simulink model "main"  (R2022a)
settings: Solver=FixedStepDiscrete  StartTime=0.0  StopTime=Inf  FixedStep=(50e-6)-(sim_en*4.995e-5)  RelTol=1e-3  EnableMultiTasking=on
model workspace (MAT data in the model file):
  Param : Simulink.Parameter (value not decoded)
  ac_ok : Simulink.Signal (value not decoded)
  ac_ok_120 : Simulink.Signal (value not decoded)
  bulk_voltage : Simulink.Signal (value not decoded)
  burstduty_integ_max : Simulink.Signal (value not decoded)
  burstduty_integ_min : Simulink.Signal (value not decoded)
  burstduty_ki : Simulink.Signal (value not decoded)
  burstduty_kp : Simulink.Signal (value not decoded)
  calib_ok : Simulink.Signal (value not decoded)
  can_addr1 : Simulink.Signal (value not decoded)
  can_addr2 : Simulink.Signal (value not decoded)
  can_addr3 : Simulink.Signal (value not decoded)
  can_addr4 : Simulink.Signal (value not decoded)
  can_data_rx : Simulink.Signal (value not decoded)
  can_data_tx : Simulink.Signal (value not decoded)
  can_timeout_120 : Simulink.Signal (value not decoded)
  chksum_scircv : Simulink.Signal (value not decoded)
  clllc_en_120 : Simulink.Signal (value not decoded)
  clllc_fault_120 : Simulink.Signal (value not decoded)
  clllc_ok_120 : Simulink.Signal (value not decoded)
  cmpss1h : Simulink.Signal (value not decoded)
  cmpss1l : Simulink.Signal (value not decoded)
  cmpss2h : Simulink.Signal (value not decoded)
  cmpss2l : Simulink.Signal (value not decoded)
  cmpss3h : Simulink.Signal (value not decoded)
  cmpss3l : Simulink.Signal (value not decoded)
  cmpss4h : Simulink.Signal (value not decoded)
  cmpss4l : Simulink.Signal (value not decoded)
  cmpss5h : Simulink.Signal (value not decoded)
  cmpss5l : Simulink.Signal (value not decoded)
  cmpss6h : Simulink.Signal (value not decoded)
  cmpss6l : Simulink.Signal (value not decoded)
  cmpss7h : Simulink.Signal (value not decoded)
  cmpss7l : Simulink.Signal (value not decoded)
  cmpss8h : Simulink.Signal (value not decoded)
  cmpss8l : Simulink.Signal (value not decoded)
  cnt_idle : Simulink.Signal (value not decoded)
  cnt_orps : Simulink.Signal (value not decoded)
  cnt_scircv : Simulink.Signal (value not decoded)
  cnt_scixmt : Simulink.Signal (value not decoded)
  cnt_scixmt_func : Simulink.Signal (value not decoded)
  cnt_temp_mux : Simulink.Signal (value not decoded)
  cnt_vdroop : Simulink.Signal (value not decoded)
  config_ok : Simulink.Signal (value not decoded)
  control_en : Simulink.Signal (value not decoded)
  cp_ready_120 : Simulink.Signal (value not decoded)
  d2d_en : Simulink.Signal (value not decoded)
  dchg_off : Simulink.Signal (value not decoded)
  debug_dacb : Simulink.Signal (value not decoded)
  debug_dacc : Simulink.Signal (value not decoded)
  debug_msg1 : Simulink.Signal (value not decoded)
  debug_msg2 : Simulink.Signal (value not decoded)
  debug_msg3 : Simulink.Signal (value not decoded)
  debug_msg4 : Simulink.Signal (value not decoded)
  debug_msg5 : Simulink.Signal (value not decoded)
  debug_msg6 : Simulink.Signal (value not decoded)
  dir_v2g : Simulink.Signal (value not decoded)
  eoss_llc1 : Simulink.Signal (value not decoded)
  eoss_llc2 : Simulink.Signal (value not decoded)
  eoss_orps : Simulink.Signal (value not decoded)
  fault_ocp : Simulink.Signal (value not decoded)
  fault_otp : Simulink.Signal (value not decoded)
  fault_ovp : Simulink.Signal (value not decoded)
  fut_en : Simulink.Signal (value not decoded)
  fwd_en_120 : Simulink.Signal (value not decoded)
  gain_llc1_sec_idc : Simulink.Signal (value not decoded)
  gain_llc1_temp_sr : Simulink.Signal (value not decoded)
  gain_llc2_sec_idc : Simulink.Signal (value not decoded)
  gain_vbat : Simulink.Signal (value not decoded)
  gain_vbulk : Simulink.Signal (value not decoded)
  gain_vout : Simulink.Signal (value not decoded)
  input_current_phasea : Simulink.Signal (value not decoded)
  input_current_phaseb : Simulink.Signal (value not decoded)
  input_current_phasec : Simulink.Signal (value not decoded)
  input_freq : Simulink.Signal (value not decoded)
  input_power : Simulink.Signal (value not decoded)
  input_voltage_phasea : Simulink.Signal (value not decoded)
  input_voltage_phaseb : Simulink.Signal (value not decoded)
  input_voltage_phasec : Simulink.Signal (value not decoded)
  ishare_arbiter : Simulink.Signal (value not decoded)
  ishare_thresh : Simulink.Signal (value not decoded)
  led_g : Simulink.Signal (value not decoded)
  led_r : Simulink.Signal (value not decoded)
  led_y : Simulink.Signal (value not decoded)
  llc1_burst_integ : Simulink.Signal (value not decoded)
  llc1_burstduty_buffer : Simulink.Signal (value not decoded)
  llc1_pfm_error : Simulink.Signal (value not decoded)
  llc1_pfm_integ : Simulink.Signal (value not decoded)
  llc1_pfm_prop : Simulink.Signal (value not decoded)
  llc1_pri_idc : Simulink.Signal (value not decoded)
  llc1_ps_buffer : Simulink.Signal (value not decoded)
  llc1_pspwm_error : Simulink.Signal (value not decoded)
  llc1_pspwm_integ : Simulink.Signal (value not decoded)
  llc1_pspwm_prop : Simulink.Signal (value not decoded)
  llc1_sec_idc : Simulink.Signal (value not decoded)
  llc1_temp_sr : Simulink.Signal (value not decoded)
  llc1_ts_tbctr_buffer : Simulink.Signal (value not decoded)
  llc2_burst_integ : Simulink.Signal (value not decoded)
  llc2_burstduty_buffer : Simulink.Signal (value not decoded)
  llc2_en : Simulink.Signal (value not decoded)
  llc2_en_buffer : Simulink.Signal (value not decoded)
  llc2_pfm_error : Simulink.Signal (value not decoded)
  llc2_pfm_integ : Simulink.Signal (value not decoded)
  llc2_pfm_prop : Simulink.Signal (value not decoded)
  llc2_pri_idc : Simulink.Signal (value not decoded)
  llc2_ps_buffer : Simulink.Signal (value not decoded)
  llc2_pspwm_error : Simulink.Signal (value not decoded)
  llc2_pspwm_integ : Simulink.Signal (value not decoded)
  llc2_pspwm_prop : Simulink.Signal (value not decoded)
  llc2_sec_idc : Simulink.Signal (value not decoded)
  llc2_temp_sr : Simulink.Signal (value not decoded)
  llc2_ts_tbctr_buffer : Simulink.Signal (value not decoded)
  loop_adcint : Simulink.Signal (value not decoded)
  loop_control : Simulink.Signal (value not decoded)
  loop_idle : Simulink.Signal (value not decoded)
  mid_bulk_voltage : Simulink.Signal (value not decoded)
  mode_120 : Simulink.Signal (value not decoded)
  mode_cc_cv : Simulink.Signal (value not decoded)
  myParam : mpt.Parameter (value not decoded)
  obc_ok_120 : Simulink.Signal (value not decoded)
  offset_llc1_sec_idc : Simulink.Signal (value not decoded)
  offset_llc1_temp_sr : Simulink.Signal (value not decoded)
  offset_llc2_sec_idc : Simulink.Signal (value not decoded)
  offset_vbat : Simulink.Signal (value not decoded)
  offset_vbulk : Simulink.Signal (value not decoded)
  offset_vout : Simulink.Signal (value not decoded)
  openloop_en : Simulink.Signal (value not decoded)
  openloop_fault_en : Simulink.Signal (value not decoded)
  ot_fault_120 : Simulink.Signal (value not decoded)
  pfc_en : Simulink.Signal (value not decoded)
  pfc_en_120 : Simulink.Signal (value not decoded)
  pfc_fw_revision : Simulink.Signal (value not decoded)
  pfc_fw_revision_bootloader : Simulink.Signal (value not decoded)
  pfc_fw_revision_debug : Simulink.Signal (value not decoded)
  pfc_ok : Simulink.Signal (value not decoded)
  pfc_ok_120 : Simulink.Signal (value not decoded)
  pfm_a0 : Simulink.Signal (value not decoded)
  pfm_a1 : Simulink.Signal (value not decoded)
  pfm_integ_max : Simulink.Signal (value not decoded)
  pfm_integ_min : Simulink.Signal (value not decoded)
  pfm_ki : Simulink.Signal (value not decoded)
  pfm_kp : Simulink.Signal (value not decoded)
  pri_fut_en : Simulink.Signal (value not decoded)
  pri_fut_en_buffer : Simulink.Signal (value not decoded)
  pri_halfbridge_en : Simulink.Signal (value not decoded)
  pri_halfbridge_en_buffer : Simulink.Signal (value not decoded)
  pspwm_integ_max : Simulink.Signal (value not decoded)
  pspwm_integ_min : Simulink.Signal (value not decoded)
  pspwm_ki : Simulink.Signal (value not decoded)
  pspwm_kp : Simulink.Signal (value not decoded)
  ref_idclink_max : Simulink.Signal (value not decoded)
  ref_iout : Simulink.Signal (value not decoded)
  ref_iout_calib : Simulink.Signal (value not decoded)
  ref_iout_llc1 : Simulink.Signal (value not decoded)
  ref_iout_llc1_calib : Simulink.Signal (value not decoded)
  ref_iout_llc2 : Simulink.Signal (value not decoded)
  ref_iout_llc2_calib : Simulink.Signal (value not decoded)
  ref_pout : Simulink.Signal (value not decoded)
  ref_ss_llc1 : Simulink.Signal (value not decoded)
  ref_ss_llc2 : Simulink.Signal (value not decoded)
  ref_ss_orps : Simulink.Signal (value not decoded)
  ref_vbat : Simulink.Signal (value not decoded)
  ref_vbat_calib : Simulink.Signal (value not decoded)
  ref_vbulk : Simulink.Signal (value not decoded)
  ref_vbulk_calib : Simulink.Signal (value not decoded)
  ref_vbulk_llc1_calib : Simulink.Signal (value not decoded)
  ref_vbulk_llc2_calib : Simulink.Signal (value not decoded)
  ref_vout : Simulink.Signal (value not decoded)
  ref_vout_calib : Simulink.Signal (value not decoded)
  relay_en : Simulink.Signal (value not decoded)
  reset_flag : Simulink.Signal (value not decoded)
  rev_en_120 : Simulink.Signal (value not decoded)
  runtime_control : Simulink.Signal (value not decoded)
  runtime_idle : Simulink.Signal (value not decoded)
  scircv_buffer : Simulink.Signal (value not decoded)
  scircv_buffer_tmp : Simulink.Signal (value not decoded)
  scircv_buffer_tmp_idx0 : Simulink.Signal (value not decoded)
  scircv_chksum : Simulink.Signal (value not decoded)
  scircv_chksum_ok : Simulink.Signal (value not decoded)
  scircv_parse_ok : Simulink.Signal (value not decoded)
  scixmt_buffer : Simulink.Signal (value not decoded)
  scixmt_chksum : Simulink.Signal (value not decoded)
  scixmt_func : Simulink.Signal (value not decoded)
  scixmt_word0_lsb : Simulink.Signal (value not decoded)
  scixmt_word0_msb : Simulink.Signal (value not decoded)
  scixmt_word1_lsb : Simulink.Signal (value not decoded)
  scixmt_word1_msb : Simulink.Signal (value not decoded)
  scixmt_word2_lsb : Simulink.Signal (value not decoded)
  scixmt_word2_msb : Simulink.Signal (value not decoded)
  scixmt_wr : Simulink.Signal (value not decoded)
  ss_step : Simulink.Signal (value not decoded)
  state_calib : Simulink.Signal (value not decoded)
  state_control : Simulink.Signal (value not decoded)
  state_hkeep : Simulink.Signal (value not decoded)
  status_cmpss : Simulink.Signal (value not decoded)
  status_control : Simulink.Signal (value not decoded)
  status_digin : Simulink.Signal (value not decoded)
  status_digout : Simulink.Signal (value not decoded)
  status_fault : Simulink.Signal (value not decoded)
  status_input : Simulink.Signal (value not decoded)
  status_pfc : Simulink.Signal (value not decoded)
  temp_inlet : Simulink.Signal (value not decoded)
  temp_llc1_fet_hs : Simulink.Signal (value not decoded)
  temp_llc2_fet_hs : Simulink.Signal (value not decoded)
  temp_mux : Simulink.Signal (value not decoded)
  temp_mux_s0 : Simulink.Signal (value not decoded)
  temp_mux_s1 : Simulink.Signal (value not decoded)
  temp_mux_s2 : Simulink.Signal (value not decoded)
  temp_outlet : Simulink.Signal (value not decoded)
  temp_pfc_fet_hsa : Simulink.Signal (value not decoded)
  temp_pfc_fet_hsb : Simulink.Signal (value not decoded)
  temp_pfc_fet_hsc : Simulink.Signal (value not decoded)
  temp_pfc_fet_lsa : Simulink.Signal (value not decoded)
  temp_pfc_fet_lsb : Simulink.Signal (value not decoded)
  temp_pfc_fet_lsc : Simulink.Signal (value not decoded)
  test_mode : Simulink.Signal (value not decoded)
  tfcv_cc : Simulink.Signal (value not decoded)
  tfcv_cc_llc2 : Simulink.Signal (value not decoded)
  tfcv_cv : Simulink.Signal (value not decoded)
  tfcv_sr_en : Simulink.Signal (value not decoded)
  tfv_assert_llc1_pri_idc : Simulink.Signal (value not decoded)
  tfv_assert_llc1_sec_idc : Simulink.Signal (value not decoded)
  tfv_assert_llc1_temp_sr : Simulink.Signal (value not decoded)
  tfv_assert_llc2_pri_idc : Simulink.Signal (value not decoded)
  tfv_assert_llc2_sec_idc : Simulink.Signal (value not decoded)
  tfv_assert_llc2_temp_sr : Simulink.Signal (value not decoded)
  tfv_assert_temp_outlet : Simulink.Signal (value not decoded)
  tfv_assert_vaux_uv : Simulink.Signal (value not decoded)
  tfv_assert_vbat : Simulink.Signal (value not decoded)
  tfv_assert_vbulk : Simulink.Signal (value not decoded)
  tfv_assert_vout : Simulink.Signal (value not decoded)
  tfv_cnt_tz : Simulink.Signal (value not decoded)
  tfv_deassert_llc1_pri_idc : Simulink.Signal (value not decoded)
  tfv_deassert_llc1_sec_idc : Simulink.Signal (value not decoded)
  tfv_deassert_llc1_temp_sr : Simulink.Signal (value not decoded)
  tfv_deassert_llc2_pri_idc : Simulink.Signal (value not decoded)
  tfv_deassert_llc2_sec_idc : Simulink.Signal (value not decoded)
  tfv_deassert_llc2_temp_sr : Simulink.Signal (value not decoded)
  tfv_deassert_temp_outlet : Simulink.Signal (value not decoded)
  tfv_deassert_vaux_uv : Simulink.Signal (value not decoded)
  tfv_deassert_vbat : Simulink.Signal (value not decoded)
  tfv_deassert_vbulk : Simulink.Signal (value not decoded)
  tfv_deassert_vout : Simulink.Signal (value not decoded)
  tfv_llc1_pri_idc : Simulink.Signal (value not decoded)
  tfv_llc1_sec_idc : Simulink.Signal (value not decoded)
  tfv_llc1_temp_sr : Simulink.Signal (value not decoded)
  tfv_llc2_pri_idc : Simulink.Signal (value not decoded)
  tfv_llc2_sec_idc : Simulink.Signal (value not decoded)
  tfv_llc2_temp_sr : Simulink.Signal (value not decoded)
  tfv_temp_outlet : Simulink.Signal (value not decoded)
  tfv_vaux_uv : Simulink.Signal (value not decoded)
  tfv_vbat : Simulink.Signal (value not decoded)
  tfv_vbulk : Simulink.Signal (value not decoded)
  tfv_vout : Simulink.Signal (value not decoded)
  timer_1ms : Simulink.Signal (value not decoded)
  tz : Simulink.Signal (value not decoded)
  valve_en : Simulink.Signal (value not decoded)
  vaux : Simulink.Signal (value not decoded)
  vbat : Simulink.Signal (value not decoded)
  vbulk : Simulink.Signal (value not decoded)
  vout : Simulink.Signal (value not decoded)
undefined symbols (not defined in the file or in its folder): CAN_O_INT, CANA_BASE, Down, GPTRIP1SEL, GPTRIP2SEL, TZ1, TZ2, Up
libraries: hdlsllib x159, simulink x94, c2802xlib x32, c2837xDlib x19, c2807xlib x16, c280xlib x13, canmsglib x8, idelinklib_common x2, c2000lib x1, c281xlib x1
(part 14 of 20)

== system main/Task_Manager/idle/idle_task/comm_npc/comm_npc/COMM_NPC.extractScircv/pfc_main_info ==
  note: Note:
      | byte0 - header
      | byte1 - w/r
      | byte2 - func
      | byte3, byte4 - word0_lsb, word0_msb
      | byte5, byte6 - word1_lsb, word1_msb
      | byte7, byte8 - word2_lsb, word2_msb
      | byte9 - chksum
      | byte10 - 0x00
      | byte11 - terminator
  scircv_buffer : Inport
  Action Port : ActionPort  ActionPortLabel=case [ 4 ]:
  Add : Sum  AccumDataTypeStr=uint16  OutDataTypeStr=uint16
  Add1 : Sum  AccumDataTypeStr=uint16  OutDataTypeStr=uint16
  Add2 : Sum  AccumDataTypeStr=uint16  OutDataTypeStr=uint16
  Bit Shift : hdlsllib/Logic and Bit Operations/Bit Shift  mode=Shift Left Logical  N=8
  Bit Shift1 : hdlsllib/Logic and Bit Operations/Bit Shift  mode=Shift Left Logical  N=8
  Bit Shift2 : hdlsllib/Logic and Bit Operations/Bit Shift  mode=Shift Left Logical  N=8
  Cast To Single{1..6} (6 alike) : DataTypeConversion  OutDataTypeStr=uint16  SaturateOnIntegerOverflow=off  RndMeth=Floor
  Constant1 : Constant  Value=3  OutDataTypeStr=uint8
  Constant2 : Constant  Value=4  OutDataTypeStr=uint8
  Constant3 : Constant  Value=7  OutDataTypeStr=uint8
  Constant4 : Constant  Value=8  OutDataTypeStr=uint8
  Constant5 : Constant  Value=5  OutDataTypeStr=uint8
  Constant6 : Constant  Value=6  OutDataTypeStr=uint8
  Data Store Write1 : DataStoreWrite  DataStoreName=status_pfc  IndexOptions=Index vector (dialog)  Indices=1  OutputSizes=1
  Data Store Write2 : DataStoreWrite  DataStoreName=mid_bulk_voltage  IndexOptions=Index vector (dialog)  Indices=1  OutputSizes=1
  Data Store Write3 : DataStoreWrite  DataStoreName=bulk_voltage  IndexOptions=Index vector (dialog)  Indices=1  OutputSizes=1
  word0_lsb : Selector  IndexMode=Zero-based  InputPortWidth=12  IndexOptions=Index vector (port)  Indices=[1 3]  OutputSizes=1
  word0_lsb1 : Selector  IndexMode=Zero-based  InputPortWidth=12  IndexOptions=Index vector (port)  Indices=[1 3]  OutputSizes=1
  word0_lsb2 : Selector  IndexMode=Zero-based  InputPortWidth=12  IndexOptions=Index vector (port)  Indices=[1 3]  OutputSizes=1
  word0_msb : Selector  IndexMode=Zero-based  InputPortWidth=12  IndexOptions=Index vector (port)  Indices=[1 3]  OutputSizes=1
  word0_msb1 : Selector  IndexMode=Zero-based  InputPortWidth=12  IndexOptions=Index vector (port)  Indices=[1 3]  OutputSizes=1
  word0_msb2 : Selector  IndexMode=Zero-based  InputPortWidth=12  IndexOptions=Index vector (port)  Indices=[1 3]  OutputSizes=1
  wires:
  [scircv_buffer] -> word0_lsb/1
  Constant1/1 -> word0_lsb/2
  word0_lsb/1 -> Cast To Single1/1
  scircv_buffer/1 -> [scircv_buffer]
  Constant2/1 -> word0_msb/2
  [scircv_buffer] -> word0_msb/1
  word0_msb/1 -> Cast To Single2/1
  Bit Shift/1 -> Add/2
  Add/1 -> Data Store Write1/1
  Cast To Single1/1 -> Add/1
  Cast To Single2/1 -> Bit Shift/1
  Cast To Single4/1 -> Bit Shift1/1
  Cast To Single3/1 -> Add1/1
  Add1/1 -> Data Store Write2/1
  Bit Shift1/1 -> Add1/2
  word0_msb1/1 -> Cast To Single4/1
  [scircv_buffer] -> word0_msb1/1
  Constant4/1 -> word0_msb1/2
  word0_lsb1/1 -> Cast To Single3/1
  Constant3/1 -> word0_lsb1/2
  [scircv_buffer] -> word0_lsb1/1
  Cast To Single6/1 -> Bit Shift2/1
  Cast To Single5/1 -> Add2/1
  Add2/1 -> Data Store Write3/1
  Bit Shift2/1 -> Add2/2
  word0_msb2/1 -> Cast To Single6/1
  [scircv_buffer] -> word0_msb2/1
  Constant6/1 -> word0_msb2/2
  word0_lsb2/1 -> Cast To Single5/1
  Constant5/1 -> word0_lsb2/2
  [scircv_buffer] -> word0_lsb2/1

== system main/Task_Manager/idle/idle_task/comm_npc/comm_npc/COMM_NPC.extractScircv/pri_debug_msga ==
  note: Note:
      | byte0 - header
      | byte1 - w/r
      | byte2 - func
      | byte3, byte4 - word0_lsb, word0_msb
      | byte5, byte6 - word1_lsb, word1_msb
      | byte7, byte8 - word2_lsb, word2_msb
      | byte9 - chksum
      | byte10 - 0x00
      | byte11 - terminator
  scircv_buffer : Inport
  Action Port : ActionPort  ActionPortLabel=case [ 49 ]:
  Add : Sum  AccumDataTypeStr=uint16  OutDataTypeStr=uint16
  Add1 : Sum  AccumDataTypeStr=uint16  OutDataTypeStr=uint16
  Add2 : Sum  AccumDataTypeStr=uint16  OutDataTypeStr=uint16
  Bit Shift : hdlsllib/Logic and Bit Operations/Bit Shift  mode=Shift Left Logical  N=8
  Bit Shift1 : hdlsllib/Logic and Bit Operations/Bit Shift  mode=Shift Left Logical  N=8
  Bit Shift2 : hdlsllib/Logic and Bit Operations/Bit Shift  mode=Shift Left Logical  N=8
  Cast To Single{1..6} (6 alike) : DataTypeConversion  OutDataTypeStr=uint16  SaturateOnIntegerOverflow=off  RndMeth=Floor
  Constant1 : Constant  Value=3  OutDataTypeStr=uint8
  Constant2 : Constant  Value=4  OutDataTypeStr=uint8
  Constant3 : Constant  Value=7  OutDataTypeStr=uint8
  Constant4 : Constant  Value=8  OutDataTypeStr=uint8
  Constant5 : Constant  Value=5  OutDataTypeStr=uint8
  Constant6 : Constant  Value=6  OutDataTypeStr=uint8
  Data Store Write1 : DataStoreWrite  DataStoreName=debug_msg1  IndexOptions=Index vector (dialog)  Indices=1  OutputSizes=1
  Data Store Write2 : DataStoreWrite  DataStoreName=debug_msg3  IndexOptions=Index vector (dialog)  Indices=1  OutputSizes=1
  Data Store Write3 : DataStoreWrite  DataStoreName=debug_msg2  IndexOptions=Index vector (dialog)  Indices=1  OutputSizes=1
  word0_lsb : Selector  IndexMode=Zero-based  InputPortWidth=12  IndexOptions=Index vector (port)  Indices=[1 3]  OutputSizes=1
  word0_lsb1 : Selector  IndexMode=Zero-based  InputPortWidth=12  IndexOptions=Index vector (port)  Indices=[1 3]  OutputSizes=1
  word0_lsb2 : Selector  IndexMode=Zero-based  InputPortWidth=12  IndexOptions=Index vector (port)  Indices=[1 3]  OutputSizes=1
  word0_msb : Selector  IndexMode=Zero-based  InputPortWidth=12  IndexOptions=Index vector (port)  Indices=[1 3]  OutputSizes=1
  word0_msb1 : Selector  IndexMode=Zero-based  InputPortWidth=12  IndexOptions=Index vector (port)  Indices=[1 3]  OutputSizes=1
  word0_msb2 : Selector  IndexMode=Zero-based  InputPortWidth=12  IndexOptions=Index vector (port)  Indices=[1 3]  OutputSizes=1
  wires:
  [scircv_buffer] -> word0_lsb2/1
  Constant5/1 -> word0_lsb2/2
  word0_lsb2/1 -> Cast To Single5/1
  Constant6/1 -> word0_msb2/2
  [scircv_buffer] -> word0_msb2/1
  word0_msb2/1 -> Cast To Single6/1
  Bit Shift2/1 -> Add2/2
  Add2/1 -> Data Store Write3/1
  Cast To Single5/1 -> Add2/1
  Cast To Single6/1 -> Bit Shift2/1
  [scircv_buffer] -> word0_lsb1/1
  Constant3/1 -> word0_lsb1/2
  word0_lsb1/1 -> Cast To Single3/1
  Constant4/1 -> word0_msb1/2
  [scircv_buffer] -> word0_msb1/1
  word0_msb1/1 -> Cast To Single4/1
  Bit Shift1/1 -> Add1/2
  Add1/1 -> Data Store Write2/1
  Cast To Single3/1 -> Add1/1
  Cast To Single4/1 -> Bit Shift1/1
  Cast To Single2/1 -> Bit Shift/1
  Cast To Single1/1 -> Add/1
  Add/1 -> Data Store Write1/1
  Bit Shift/1 -> Add/2
  word0_msb/1 -> Cast To Single2/1
  [scircv_buffer] -> word0_msb/1
  Constant2/1 -> word0_msb/2
  scircv_buffer/1 -> [scircv_buffer]
  word0_lsb/1 -> Cast To Single1/1
  Constant1/1 -> word0_lsb/2
  [scircv_buffer] -> word0_lsb/1

== system main/Task_Manager/idle/idle_task/comm_npc/comm_npc/COMM_NPC.extractScircv/pri_debug_msgb ==
  note: Note:
      | byte0 - header
      | byte1 - w/r
      | byte2 - func
      | byte3, byte4 - word0_lsb, word0_msb
      | byte5, byte6 - word1_lsb, word1_msb
      | byte7, byte8 - word2_lsb, word2_msb
      | byte9 - chksum
      | byte10 - 0x00
      | byte11 - terminator
  scircv_buffer : Inport
  Action Port : ActionPort  ActionPortLabel=case [ 50 ]:
  Add : Sum  AccumDataTypeStr=uint16  OutDataTypeStr=uint16
  Add1 : Sum  AccumDataTypeStr=uint16  OutDataTypeStr=uint16
  Add2 : Sum  AccumDataTypeStr=uint16  OutDataTypeStr=uint16
  Bit Shift : hdlsllib/Logic and Bit Operations/Bit Shift  mode=Shift Left Logical  N=8
  Bit Shift1 : hdlsllib/Logic and Bit Operations/Bit Shift  mode=Shift Left Logical  N=8
  Bit Shift2 : hdlsllib/Logic and Bit Operations/Bit Shift  mode=Shift Left Logical  N=8
  Cast To Single{1..6} (6 alike) : DataTypeConversion  OutDataTypeStr=uint16  SaturateOnIntegerOverflow=off  RndMeth=Floor
  Constant1 : Constant  Value=3  OutDataTypeStr=uint8
  Constant2 : Constant  Value=4  OutDataTypeStr=uint8
  Constant3 : Constant  Value=7  OutDataTypeStr=uint8
  Constant4 : Constant  Value=8  OutDataTypeStr=uint8
  Constant5 : Constant  Value=5  OutDataTypeStr=uint8
  Constant6 : Constant  Value=6  OutDataTypeStr=uint8
  Data Store Write1 : DataStoreWrite  DataStoreName=debug_msg4  IndexOptions=Index vector (dialog)  Indices=1  OutputSizes=1
  Data Store Write2 : DataStoreWrite  DataStoreName=debug_msg6  IndexOptions=Index vector (dialog)  Indices=1  OutputSizes=1
  Data Store Write3 : DataStoreWrite  DataStoreName=debug_msg5  IndexOptions=Index vector (dialog)  Indices=1  OutputSizes=1
  word0_lsb : Selector  IndexMode=Zero-based  InputPortWidth=12  IndexOptions=Index vector (port)  Indices=[1 3]  OutputSizes=1
  word0_lsb1 : Selector  IndexMode=Zero-based  InputPortWidth=12  IndexOptions=Index vector (port)  Indices=[1 3]  OutputSizes=1
  word0_lsb2 : Selector  IndexMode=Zero-based  InputPortWidth=12  IndexOptions=Index vector (port)  Indices=[1 3]  OutputSizes=1
  word0_msb : Selector  IndexMode=Zero-based  InputPortWidth=12  IndexOptions=Index vector (port)  Indices=[1 3]  OutputSizes=1
  word0_msb1 : Selector  IndexMode=Zero-based  InputPortWidth=12  IndexOptions=Index vector (port)  Indices=[1 3]  OutputSizes=1
  word0_msb2 : Selector  IndexMode=Zero-based  InputPortWidth=12  IndexOptions=Index vector (port)  Indices=[1 3]  OutputSizes=1
  wires:
  [scircv_buffer] -> word0_lsb/1
  Constant1/1 -> word0_lsb/2
  word0_lsb/1 -> Cast To Single1/1
  scircv_buffer/1 -> [scircv_buffer]
  Constant2/1 -> word0_msb/2
  [scircv_buffer] -> word0_msb/1
  word0_msb/1 -> Cast To Single2/1
  Bit Shift/1 -> Add/2
  Add/1 -> Data Store Write1/1
  Cast To Single1/1 -> Add/1
  Cast To Single2/1 -> Bit Shift/1
  Cast To Single4/1 -> Bit Shift1/1
  Cast To Single3/1 -> Add1/1
  Add1/1 -> Data Store Write2/1
  Bit Shift1/1 -> Add1/2
  word0_msb1/1 -> Cast To Single4/1
  [scircv_buffer] -> word0_msb1/1
  Constant4/1 -> word0_msb1/2
  word0_lsb1/1 -> Cast To Single3/1
  Constant3/1 -> word0_lsb1/2
  [scircv_buffer] -> word0_lsb1/1
  Cast To Single6/1 -> Bit Shift2/1
  Cast To Single5/1 -> Add2/1
  Add2/1 -> Data Store Write3/1
  Bit Shift2/1 -> Add2/2
  word0_msb2/1 -> Cast To Single6/1
  [scircv_buffer] -> word0_msb2/1
  Constant6/1 -> word0_msb2/2
  word0_lsb2/1 -> Cast To Single5/1
  Constant5/1 -> word0_lsb2/2
  [scircv_buffer] -> word0_lsb2/1

== system main/Task_Manager/idle/idle_task/comm_npc/comm_npc/COMM_NPC.extractScircv/pri_fut_en ==
  note: Note:
      | byte0 - header
      | byte1 - w/r
      | byte2 - func
      | byte3, byte4 - word0_lsb, word0_msb
      | byte5, byte6 - word1_lsb, word1_msb
      | byte7, byte8 - word2_lsb, word2_msb
      | byte9 - chksum
      | byte10 - 0x00
      | byte11 - terminator
  scircv_buffer : Inport
  Action Port : ActionPort  ActionPortLabel=case [ 33 ]:
  Cast To Single3 : DataTypeConversion  OutDataTypeStr=uint16  SaturateOnIntegerOverflow=off  RndMeth=Floor
  Constant1 : Constant  Value=3  OutDataTypeStr=uint8
  Data Store Write1 : DataStoreWrite  DataStoreName=pri_fut_en  IndexOptions=Index vector (dialog)  Indices=1  OutputSizes=1
  word0_lsb : Selector  IndexMode=Zero-based  InputPortWidth=12  IndexOptions=Index vector (port)  Indices=[1 3]  OutputSizes=1
  wires:
  Cast To Single3/1 -> Data Store Write1/1
  scircv_buffer/1 -> [scircv_buffer]
  word0_lsb/1 -> Cast To Single3/1
  Constant1/1 -> word0_lsb/2
  [scircv_buffer] -> word0_lsb/1

== system main/Task_Manager/idle/idle_task/comm_npc/comm_npc/COMM_NPC.extractScircv/pri_temp_info1 ==
  note: Note:
      | byte0 - header
      | byte1 - w/r
      | byte2 - func
      | byte3, byte4 - word0_lsb, word0_msb
      | byte5, byte6 - word1_lsb, word1_msb
      | byte7, byte8 - word2_lsb, word2_msb
      | byte9 - chksum
      | byte10 - 0x00
      | byte11 - terminator
  scircv_buffer : Inport
  Action Port : ActionPort  ActionPortLabel=case [ 6 ]:
  Add : Sum  AccumDataTypeStr=uint16  OutDataTypeStr=uint16
  Add1 : Sum  AccumDataTypeStr=uint16  OutDataTypeStr=uint16
  Add2 : Sum  AccumDataTypeStr=uint16  OutDataTypeStr=uint16
  Bit Shift : hdlsllib/Logic and Bit Operations/Bit Shift  mode=Shift Left Logical  N=8
  Bit Shift1 : hdlsllib/Logic and Bit Operations/Bit Shift  mode=Shift Left Logical  N=8
  Bit Shift2 : hdlsllib/Logic and Bit Operations/Bit Shift  mode=Shift Left Logical  N=8
  Cast To Single{1..6} (6 alike) : DataTypeConversion  OutDataTypeStr=uint16  SaturateOnIntegerOverflow=off  RndMeth=Floor
  Constant1 : Constant  Value=3  OutDataTypeStr=uint8
  Constant2 : Constant  Value=4  OutDataTypeStr=uint8
  Constant3 : Constant  Value=7  OutDataTypeStr=uint8
  Constant4 : Constant  Value=8  OutDataTypeStr=uint8
  Constant5 : Constant  Value=5  OutDataTypeStr=uint8
  Constant6 : Constant  Value=6  OutDataTypeStr=uint8
  Data Store Write1 : DataStoreWrite  DataStoreName=temp_pfc_fet_hsa  IndexOptions=Index vector (dialog)  Indices=1  OutputSizes=1
  Data Store Write2 : DataStoreWrite  DataStoreName=temp_pfc_fet_hsb  IndexOptions=Index vector (dialog)  Indices=1  OutputSizes=1
  Data Store Write3 : DataStoreWrite  DataStoreName=temp_pfc_fet_lsa  IndexOptions=Index vector (dialog)  Indices=1  OutputSizes=1
  word0_lsb : Selector  IndexMode=Zero-based  InputPortWidth=12  IndexOptions=Index vector (port)  Indices=[1 3]  OutputSizes=1
  word0_lsb1 : Selector  IndexMode=Zero-based  InputPortWidth=12  IndexOptions=Index vector (port)  Indices=[1 3]  OutputSizes=1
  word0_lsb2 : Selector  IndexMode=Zero-based  InputPortWidth=12  IndexOptions=Index vector (port)  Indices=[1 3]  OutputSizes=1
  word0_msb : Selector  IndexMode=Zero-based  InputPortWidth=12  IndexOptions=Index vector (port)  Indices=[1 3]  OutputSizes=1
  word0_msb1 : Selector  IndexMode=Zero-based  InputPortWidth=12  IndexOptions=Index vector (port)  Indices=[1 3]  OutputSizes=1
  word0_msb2 : Selector  IndexMode=Zero-based  InputPortWidth=12  IndexOptions=Index vector (port)  Indices=[1 3]  OutputSizes=1
  wires:
  [scircv_buffer] -> word0_lsb/1
  Constant1/1 -> word0_lsb/2
  word0_lsb/1 -> Cast To Single1/1
  scircv_buffer/1 -> [scircv_buffer]
  Constant2/1 -> word0_msb/2
  [scircv_buffer] -> word0_msb/1
  word0_msb/1 -> Cast To Single2/1
  Bit Shift/1 -> Add/2
  Add/1 -> Data Store Write1/1
  Cast To Single1/1 -> Add/1
  Cast To Single2/1 -> Bit Shift/1
  Cast To Single4/1 -> Bit Shift1/1
  Cast To Single3/1 -> Add1/1
  Add1/1 -> Data Store Write2/1
  Bit Shift1/1 -> Add1/2
  word0_msb1/1 -> Cast To Single4/1
  [scircv_buffer] -> word0_msb1/1
  Constant4/1 -> word0_msb1/2
  word0_lsb1/1 -> Cast To Single3/1
  Constant3/1 -> word0_lsb1/2
  [scircv_buffer] -> word0_lsb1/1
  Cast To Single6/1 -> Bit Shift2/1
  Cast To Single5/1 -> Add2/1
  Add2/1 -> Data Store Write3/1
  Bit Shift2/1 -> Add2/2
  word0_msb2/1 -> Cast To Single6/1
  [scircv_buffer] -> word0_msb2/1
  Constant6/1 -> word0_msb2/2
  word0_lsb2/1 -> Cast To Single5/1
  Constant5/1 -> word0_lsb2/2
  [scircv_buffer] -> word0_lsb2/1

== system main/Task_Manager/idle/idle_task/comm_npc/comm_npc/COMM_NPC.extractScircv/pri_temp_info2 ==
  note: Note:
      | byte0 - header
      | byte1 - w/r
      | byte2 - func
      | byte3, byte4 - word0_lsb, word0_msb
      | byte5, byte6 - word1_lsb, word1_msb
      | byte7, byte8 - word2_lsb, word2_msb
      | byte9 - chksum
      | byte10 - 0x00
      | byte11 - terminator
  scircv_buffer : Inport
  Action Port : ActionPort  ActionPortLabel=case [ 7 ]:
  Add : Sum  AccumDataTypeStr=uint16  OutDataTypeStr=uint16
  Add1 : Sum  AccumDataTypeStr=uint16  OutDataTypeStr=uint16
  Add2 : Sum  AccumDataTypeStr=uint16  OutDataTypeStr=uint16
  Bit Shift : hdlsllib/Logic and Bit Operations/Bit Shift  mode=Shift Left Logical  N=8
  Bit Shift1 : hdlsllib/Logic and Bit Operations/Bit Shift  mode=Shift Left Logical  N=8
  Bit Shift2 : hdlsllib/Logic and Bit Operations/Bit Shift  mode=Shift Left Logical  N=8
  Cast To Single{1..6} (6 alike) : DataTypeConversion  OutDataTypeStr=uint16  SaturateOnIntegerOverflow=off  RndMeth=Floor
  Constant1 : Constant  Value=3  OutDataTypeStr=uint8
  Constant2 : Constant  Value=4  OutDataTypeStr=uint8
  Constant3 : Constant  Value=7  OutDataTypeStr=uint8
  Constant4 : Constant  Value=8  OutDataTypeStr=uint8
  Constant5 : Constant  Value=5  OutDataTypeStr=uint8
  Constant6 : Constant  Value=6  OutDataTypeStr=uint8
  Data Store Write1 : DataStoreWrite  DataStoreName=temp_pfc_fet_lsb  IndexOptions=Index vector (dialog)  Indices=1  OutputSizes=1
  Data Store Write2 : DataStoreWrite  DataStoreName=temp_pfc_fet_lsc  IndexOptions=Index vector (dialog)  Indices=1  OutputSizes=1
  Data Store Write3 : DataStoreWrite  DataStoreName=temp_pfc_fet_hsc  IndexOptions=Index vector (dialog)  Indices=1  OutputSizes=1
  word0_lsb : Selector  IndexMode=Zero-based  InputPortWidth=12  IndexOptions=Index vector (port)  Indices=[1 3]  OutputSizes=1
  word0_lsb1 : Selector  IndexMode=Zero-based  InputPortWidth=12  IndexOptions=Index vector (port)  Indices=[1 3]  OutputSizes=1
  word0_lsb2 : Selector  IndexMode=Zero-based  InputPortWidth=12  IndexOptions=Index vector (port)  Indices=[1 3]  OutputSizes=1
  word0_msb : Selector  IndexMode=Zero-based  InputPortWidth=12  IndexOptions=Index vector (port)  Indices=[1 3]  OutputSizes=1
  word0_msb1 : Selector  IndexMode=Zero-based  InputPortWidth=12  IndexOptions=Index vector (port)  Indices=[1 3]  OutputSizes=1
  word0_msb2 : Selector  IndexMode=Zero-based  InputPortWidth=12  IndexOptions=Index vector (port)  Indices=[1 3]  OutputSizes=1
  wires:
  [scircv_buffer] -> word0_lsb/1
  Constant1/1 -> word0_lsb/2
  word0_lsb/1 -> Cast To Single1/1
  scircv_buffer/1 -> [scircv_buffer]
  Constant2/1 -> word0_msb/2
  [scircv_buffer] -> word0_msb/1
  word0_msb/1 -> Cast To Single2/1
  Bit Shift/1 -> Add/2
  Add/1 -> Data Store Write1/1
  Cast To Single1/1 -> Add/1
  Cast To Single2/1 -> Bit Shift/1
  Cast To Single4/1 -> Bit Shift1/1
  Cast To Single3/1 -> Add1/1
  Add1/1 -> Data Store Write2/1
  Bit Shift1/1 -> Add1/2
  word0_msb1/1 -> Cast To Single4/1
  [scircv_buffer] -> word0_msb1/1
  Constant4/1 -> word0_msb1/2
  word0_lsb1/1 -> Cast To Single3/1
  Constant3/1 -> word0_lsb1/2
  [scircv_buffer] -> word0_lsb1/1
  Cast To Single6/1 -> Bit Shift2/1
  Cast To Single5/1 -> Add2/1
  Add2/1 -> Data Store Write3/1
  Bit Shift2/1 -> Add2/2
  word0_msb2/1 -> Cast To Single6/1
  [scircv_buffer] -> word0_msb2/1
  Constant6/1 -> word0_msb2/2
  word0_lsb2/1 -> Cast To Single5/1
  Constant5/1 -> word0_lsb2/2
  [scircv_buffer] -> word0_lsb2/1

== system main/Task_Manager/idle/idle_task/comm_npc/comm_npc/COMM_NPC.extractScircv/pri_temp_info3 ==
  note: Note:
      | byte0 - header
      | byte1 - w/r
      | byte2 - func
      | byte3, byte4 - word0_lsb, word0_msb
      | byte5, byte6 - word1_lsb, word1_msb
      | byte7, byte8 - word2_lsb, word2_msb
      | byte9 - chksum
      | byte10 - 0x00
      | byte11 - terminator
  scircv_buffer : Inport
  Action Port : ActionPort  ActionPortLabel=case [ 8 ]:
  Add : Sum  AccumDataTypeStr=uint16  OutDataTypeStr=uint16
  Add1 : Sum  Commented=on  AccumDataTypeStr=uint16  OutDataTypeStr=uint16
  Add2 : Sum  AccumDataTypeStr=uint16  OutDataTypeStr=uint16
  Bit Shift : hdlsllib/Logic and Bit Operations/Bit Shift  mode=Shift Left Logical  N=8
  Bit Shift1 : hdlsllib/Logic and Bit Operations/Bit Shift  Commented=on  mode=Shift Left Logical  N=8
  Bit Shift2 : hdlsllib/Logic and Bit Operations/Bit Shift  mode=Shift Left Logical  N=8
  Cast To Single{1..2,5..6} (4 alike) : DataTypeConversion  OutDataTypeStr=uint16  SaturateOnIntegerOverflow=off  RndMeth=Floor
  Cast To Single3 : DataTypeConversion  Commented=on  OutDataTypeStr=uint16  SaturateOnIntegerOverflow=off  RndMeth=Floor
  Cast To Single4 : DataTypeConversion  Commented=on  OutDataTypeStr=uint16  SaturateOnIntegerOverflow=off  RndMeth=Floor
  Constant1 : Constant  Value=3  OutDataTypeStr=uint8
  Constant2 : Constant  Value=4  OutDataTypeStr=uint8
  Constant3 : Constant  Commented=on  Value=7  OutDataTypeStr=uint8
  Constant4 : Constant  Commented=on  Value=8  OutDataTypeStr=uint8
  Constant5 : Constant  Value=5  OutDataTypeStr=uint8
  Constant6 : Constant  Value=6  OutDataTypeStr=uint8
  Data Store Write1 : DataStoreWrite  DataStoreName=temp_llc1_fet_hs  IndexOptions=Index vector (dialog)  Indices=1  OutputSizes=1
  Data Store Write2 : DataStoreWrite  Commented=on  DataStoreName=input_phasec_voltage  IndexOptions=Index vector (dialog)  Indices=1  OutputSizes=1
  Data Store Write3 : DataStoreWrite  DataStoreName=temp_llc2_fet_hs  IndexOptions=Index vector (dialog)  Indices=1  OutputSizes=1
  From2 : From  Commented=on  GotoTag=scircv_buffer
  From3 : From  Commented=on  GotoTag=scircv_buffer
  word0_lsb : Selector  IndexMode=Zero-based  InputPortWidth=12  IndexOptions=Index vector (port)  Indices=[1 3]  OutputSizes=1
  word0_lsb1 : Selector  Commented=on  IndexMode=Zero-based  InputPortWidth=12  IndexOptions=Index vector (port)  Indices=[1 3]  OutputSizes=1
  word0_lsb2 : Selector  IndexMode=Zero-based  InputPortWidth=12  IndexOptions=Index vector (port)  Indices=[1 3]  OutputSizes=1
  word0_msb : Selector  IndexMode=Zero-based  InputPortWidth=12  IndexOptions=Index vector (port)  Indices=[1 3]  OutputSizes=1
  word0_msb1 : Selector  Commented=on  IndexMode=Zero-based  InputPortWidth=12  IndexOptions=Index vector (port)  Indices=[1 3]  OutputSizes=1
  word0_msb2 : Selector  IndexMode=Zero-based  InputPortWidth=12  IndexOptions=Index vector (port)  Indices=[1 3]  OutputSizes=1
  wires:
  [scircv_buffer] -> word0_lsb2/1
  Constant5/1 -> word0_lsb2/2
  word0_lsb2/1 -> Cast To Single5/1
  Constant6/1 -> word0_msb2/2
  [scircv_buffer] -> word0_msb2/1
  word0_msb2/1 -> Cast To Single6/1
  Bit Shift2/1 -> Add2/2
  Add2/1 -> Data Store Write3/1
  Cast To Single5/1 -> Add2/1
  Cast To Single6/1 -> Bit Shift2/1
  From2/1 -> word0_lsb1/1
  Constant3/1 -> word0_lsb1/2
  word0_lsb1/1 -> Cast To Single3/1
  Constant4/1 -> word0_msb1/2
  From3/1 -> word0_msb1/1
  word0_msb1/1 -> Cast To Single4/1
  Bit Shift1/1 -> Add1/2
  Add1/1 -> Data Store Write2/1
  Cast To Single3/1 -> Add1/1
  Cast To Single4/1 -> Bit Shift1/1
  Cast To Single2/1 -> Bit Shift/1
  Cast To Single1/1 -> Add/1
  Add/1 -> Data Store Write1/1
  Bit Shift/1 -> Add/2
  word0_msb/1 -> Cast To Single2/1
  [scircv_buffer] -> word0_msb/1
  Constant2/1 -> word0_msb/2
  scircv_buffer/1 -> [scircv_buffer]
  word0_lsb/1 -> Cast To Single1/1
  Constant1/1 -> word0_lsb/2
  [scircv_buffer] -> word0_lsb/1

== system main/Task_Manager/idle/idle_task/comm_npc/comm_npc/COMM_NPC.extractScircv/pri_temp_info4 ==
  note: Note:
      | byte0 - header
      | byte1 - w/r
      | byte2 - func
      | byte3, byte4 - word0_lsb, word0_msb
      | byte5, byte6 - word1_lsb, word1_msb
      | byte7, byte8 - word2_lsb, word2_msb
      | byte9 - chksum
      | byte10 - 0x00
      | byte11 - terminator
  scircv_buffer : Inport
  Action Port : ActionPort  ActionPortLabel=case [ 9 ]:
  Add : Sum  Commented=on  AccumDataTypeStr=uint16  OutDataTypeStr=uint16
  Add1 : Sum  Commented=on  AccumDataTypeStr=uint16  OutDataTypeStr=uint16
  Add2 : Sum  AccumDataTypeStr=uint16  OutDataTypeStr=uint16
  Bit Shift : hdlsllib/Logic and Bit Operations/Bit Shift  Commented=on  mode=Shift Left Logical  N=8
  Bit Shift1 : hdlsllib/Logic and Bit Operations/Bit Shift  Commented=on  mode=Shift Left Logical  N=8
  Bit Shift2 : hdlsllib/Logic and Bit Operations/Bit Shift  mode=Shift Left Logical  N=8
  Cast To Single{1..4} (4 alike) : DataTypeConversion  Commented=on  OutDataTypeStr=uint16  SaturateOnIntegerOverflow=off  RndMeth=Floor
  Cast To Single5 : DataTypeConversion  OutDataTypeStr=uint16  SaturateOnIntegerOverflow=off  RndMeth=Floor
  Cast To Single6 : DataTypeConversion  OutDataTypeStr=uint16  SaturateOnIntegerOverflow=off  RndMeth=Floor
  Constant1 : Constant  Commented=on  Value=3  OutDataTypeStr=uint8
  Constant2 : Constant  Commented=on  Value=4  OutDataTypeStr=uint8
  Constant3 : Constant  Commented=on  Value=7  OutDataTypeStr=uint8
  Constant4 : Constant  Commented=on  Value=8  OutDataTypeStr=uint8
  Constant5 : Constant  Value=5  OutDataTypeStr=uint8
  Constant6 : Constant  Value=6  OutDataTypeStr=uint8
  Data Store Write1 : DataStoreWrite  Commented=on  DataStoreName=input_phasea_voltage  IndexOptions=Index vector (dialog)  Indices=1  OutputSizes=1
  Data Store Write2 : DataStoreWrite  Commented=on  DataStoreName=input_phasec_voltage  IndexOptions=Index vector (dialog)  Indices=1  OutputSizes=1
  Data Store Write3 : DataStoreWrite  DataStoreName=temp_inlet  IndexOptions=Index vector (dialog)  Indices=1  OutputSizes=1
  From{,1..3} (4 alike) : From  Commented=on  GotoTag=scircv_buffer
  word0_lsb : Selector  Commented=on  IndexMode=Zero-based  InputPortWidth=12  IndexOptions=Index vector (port)  Indices=[1 3]  OutputSizes=1
  word0_lsb1 : Selector  Commented=on  IndexMode=Zero-based  InputPortWidth=12  IndexOptions=Index vector (port)  Indices=[1 3]  OutputSizes=1
  word0_lsb2 : Selector  IndexMode=Zero-based  InputPortWidth=12  IndexOptions=Index vector (port)  Indices=[1 3]  OutputSizes=1
  word0_msb : Selector  Commented=on  IndexMode=Zero-based  InputPortWidth=12  IndexOptions=Index vector (port)  Indices=[1 3]  OutputSizes=1
  word0_msb1 : Selector  Commented=on  IndexMode=Zero-based  InputPortWidth=12  IndexOptions=Index vector (port)  Indices=[1 3]  OutputSizes=1
  word0_msb2 : Selector  IndexMode=Zero-based  InputPortWidth=12  IndexOptions=Index vector (port)  Indices=[1 3]  OutputSizes=1
  wires:
  From/1 -> word0_lsb/1
  Constant1/1 -> word0_lsb/2
  word0_lsb/1 -> Cast To Single1/1
  scircv_buffer/1 -> [scircv_buffer]
  Constant2/1 -> word0_msb/2
  From1/1 -> word0_msb/1
  word0_msb/1 -> Cast To Single2/1
  Bit Shift/1 -> Add/2
  Add/1 -> Data Store Write1/1
  Cast To Single1/1 -> Add/1
  Cast To Single2/1 -> Bit Shift/1
  Cast To Single4/1 -> Bit Shift1/1
  Cast To Single3/1 -> Add1/1
  Add1/1 -> Data Store Write2/1
  Bit Shift1/1 -> Add1/2
  word0_msb1/1 -> Cast To Single4/1
  From3/1 -> word0_msb1/1
  Constant4/1 -> word0_msb1/2
  word0_lsb1/1 -> Cast To Single3/1
  Constant3/1 -> word0_lsb1/2
  From2/1 -> word0_lsb1/1
  Cast To Single6/1 -> Bit Shift2/1
  Cast To Single5/1 -> Add2/1
  Add2/1 -> Data Store Write3/1
  Bit Shift2/1 -> Add2/2
  word0_msb2/1 -> Cast To Single6/1
  [scircv_buffer] -> word0_msb2/1
  Constant6/1 -> word0_msb2/2
  word0_lsb2/1 -> Cast To Single5/1
  Constant5/1 -> word0_lsb2/2
  [scircv_buffer] -> word0_lsb2/1

== system main/Task_Manager/idle/idle_task/comm_npc/comm_npc/COMM_NPC.incrFunc/increment ==
  Action Port : ActionPort  ActionPortLabel=if(u1 < 11)
  Add : Sum  OutDataTypeStr=uint8
  Constant : Constant  OutDataTypeStr=uint8
  Data Store Read1 : DataStoreRead  DataStoreName=cnt_scixmt_func  IndexOptions=Index vector (dialog)  Indices=1  OutputSizes=1
  Data Store Write : DataStoreWrite  DataStoreName=cnt_scixmt_func  IndexOptions=Index vector (dialog)  Indices=1  OutputSizes=1
  Out1 : Outport
  wires:
  Add/1 -> Out1/1, Data Store Write/1
  Data Store Read1/1 -> Add/1
  Constant/1 -> Add/2

== system main/Task_Manager/idle/idle_task/comm_npc/comm_npc/COMM_NPC.incrFunc/saturation ==
  Action Port : ActionPort  ActionPortLabel=else
  Constant : Constant  Value=0  OutDataTypeStr=uint8
  Data Store Write : DataStoreWrite  DataStoreName=cnt_scixmt_func  IndexOptions=Index vector (dialog)  Indices=1  OutputSizes=1
  Out1 : Outport
  wires:
  Constant/1 -> Data Store Write/1, Out1/1

== system main/Task_Manager/idle/idle_task/comm_npc/comm_npc/COMM_NPC.parseScircv/For Iterator Subsystem ==
  scircv_buffer_tmp : Inport
  For Iterator : ForIterator  IterationLimit=24  IndexMode=Zero-based  IterationVariableDataType=uint8
  If : If  NumInputs=2  IfExpression=(u1 == 102) & (u2 < 13)
  Selector : Selector  IndexMode=Zero-based  InputPortWidth=24  IndexOptions=Index vector (port)  Indices=[1 3]  OutputSizes=1
  header_found_before_bit13 : Subsystem  TreatAsAtomicUnit=on
  scircv_parse_ok : Outport  InitialOutput=[0]
  wires:
  For Iterator/1 -> Selector/2, header_found_before_bit13/1(scircv_buffer_tmp_idx0), If/2
  scircv_buffer_tmp/1 -> Selector/1
  Selector/1 -> If/1
  If/1 -> header_found_before_bit13/Action
  header_found_before_bit13/1(Out1) -> scircv_parse_ok/1

== system main/Task_Manager/idle/idle_task/comm_npc/comm_npc/COMM_NPC.verifyScircvChksum/If Action Subsystem ==
  Action Port : ActionPort  ActionPortLabel=if(u1 == u2)
  Constant : Constant  OutDataTypeStr=boolean
  Outport : Outport
  wires:
  Constant/1 -> Outport/1

== system main/Task_Manager/idle/idle_task/comm_npc/comm_npc/COMM_NPC.verifyScircvChksum/If Action Subsystem1 ==
  Action Port : ActionPort  ActionPortLabel=else
  Constant : Constant  Value=0  OutDataTypeStr=boolean
  Outport : Outport
  wires:
  Constant/1 -> Outport/1

== system main/Task_Manager/idle/idle_task/hkeep/tfv/hkeep/HKEEP.tfvLlc1PriIdc ==
  input : Inport  OutDataTypeStr=uint16  PortDimensions=1
  assert_lim : Inport  Port=2  OutDataTypeStr=uint16  PortDimensions=1
  assert_vld : Inport  Port=3  OutDataTypeStr=uint16  PortDimensions=1
  deassert_lim : Inport  Port=4  OutDataTypeStr=uint16  PortDimensions=1
  deassert_vld : Inport  Port=5  OutDataTypeStr=uint16  PortDimensions=1
  f : TriggerPort  TriggerType=function-call  VariantControl=(inherit)
      settings: CopyFcn=Stateflow.SLINSF.SimulinkMan.removeBlockPreDeleteFcn  PreDeleteFcn=Stateflow.SLINSF.SimulinkMan.unsafePredeleteFcn
  Data Store Read : DataStoreRead  DataStoreName=timer_1ms  IndexOptions=Index vector (dialog)  Indices=1  OutputSizes=1
  Data Type Conversion : DataTypeConversion  OutDataTypeStr=boolean  SaturateOnIntegerOverflow=off  RndMeth=Floor
  MATLAB System : MATLABSystem  System=tfv_latch  SimulateUsing=Code generation
      mask Type: tfv_latch
      mask Display:
      | disp('tfv_latch');
      | port_label('input',1,'input');
      | port_label('input',2,'assert_lim');
      | port_label('input',3,'assert_vld');
      | port_label('input',4,'deassert_lim');
      | port_label('input',5,'deassert_vld');
      | port_label('input',6,'tmr');
      | port_label('output',1,'status');
  tfv_status : Outport  OutDataTypeStr=boolean
  wires:
  MATLAB System/1 -> Data Type Conversion/1
  Data Store Read/1 -> MATLAB System/6
  deassert_lim/1 -> MATLAB System/4
  assert_lim/1 -> MATLAB System/2
  assert_vld/1 -> MATLAB System/3
  input/1 -> MATLAB System/1
  deassert_vld/1 -> MATLAB System/5
  Data Type Conversion/1 -> tfv_status/1

== system main/Task_Manager/idle/idle_task/hkeep/tfv/hkeep/HKEEP.tfvLlc1SecIdc ==
  input : Inport  OutDataTypeStr=uint16  PortDimensions=1
  assert_lim : Inport  Port=2  OutDataTypeStr=uint16  PortDimensions=1
  assert_vld : Inport  Port=3  OutDataTypeStr=uint16  PortDimensions=1
  deassert_lim : Inport  Port=4  OutDataTypeStr=uint16  PortDimensions=1
  deassert_vld : Inport  Port=5  OutDataTypeStr=uint16  PortDimensions=1
  f : TriggerPort  TriggerType=function-call  VariantControl=(inherit)
      settings: CopyFcn=Stateflow.SLINSF.SimulinkMan.removeBlockPreDeleteFcn  PreDeleteFcn=Stateflow.SLINSF.SimulinkMan.unsafePredeleteFcn
  Data Store Read : DataStoreRead  DataStoreName=timer_1ms  IndexOptions=Index vector (dialog)  Indices=1  OutputSizes=1
  Data Type Conversion : DataTypeConversion  OutDataTypeStr=boolean  SaturateOnIntegerOverflow=off  RndMeth=Floor
  MATLAB System : MATLABSystem  System=tfv_latch  SimulateUsing=Code generation
      mask Type: tfv_latch
      mask Display:
      | disp('tfv_latch');
      | port_label('input',1,'input');
      | port_label('input',2,'assert_lim');
      | port_label('input',3,'assert_vld');
      | port_label('input',4,'deassert_lim');
      | port_label('input',5,'deassert_vld');
      | port_label('input',6,'tmr');
      | port_label('output',1,'status');
  tfv_status : Outport  OutDataTypeStr=boolean
  wires:
  MATLAB System/1 -> Data Type Conversion/1
  Data Store Read/1 -> MATLAB System/6
  deassert_lim/1 -> MATLAB System/4
  assert_lim/1 -> MATLAB System/2
  assert_vld/1 -> MATLAB System/3
  input/1 -> MATLAB System/1
  deassert_vld/1 -> MATLAB System/5
  Data Type Conversion/1 -> tfv_status/1

== system main/Task_Manager/idle/idle_task/hkeep/tfv/hkeep/HKEEP.tfvLlc1TempSr ==
  input : Inport  OutDataTypeStr=uint16
  assert_lim : Inport  Port=2  OutDataTypeStr=uint16
  assert_vld : Inport  Port=3  OutDataTypeStr=uint16
  deassert_lim : Inport  Port=4  OutDataTypeStr=uint16
  deassert_vld : Inport  Port=5  OutDataTypeStr=uint16
  f : TriggerPort  TriggerType=function-call  VariantControl=(inherit)
      settings: CopyFcn=Stateflow.SLINSF.SimulinkMan.removeBlockPreDeleteFcn  PreDeleteFcn=Stateflow.SLINSF.SimulinkMan.unsafePredeleteFcn
  Data Store Read1 : DataStoreRead  DataStoreName=timer_1ms  IndexOptions=Index vector (dialog)  Indices=1  OutputSizes=1
  Data Type Conversion : DataTypeConversion  OutDataTypeStr=boolean  SaturateOnIntegerOverflow=off  RndMeth=Floor
  MATLAB System : MATLABSystem  System=tfv_latch  SimulateUsing=Code generation
      mask Type: tfv_latch
      mask Display:
      | disp('tfv_latch');
      | port_label('input',1,'input');
      | port_label('input',2,'assert_lim');
      | port_label('input',3,'assert_vld');
      | port_label('input',4,'deassert_lim');
      | port_label('input',5,'deassert_vld');
      | port_label('input',6,'tmr');
      | port_label('output',1,'status');
  Rate Transition1 : RateTransition  Deterministic=off
  tfv_status : Outport  OutDataTypeStr=boolean  PortDimensions=1
  wires:
  MATLAB System/1 -> Data Type Conversion/1
  deassert_vld/1 -> MATLAB System/5
  Data Store Read1/1 -> MATLAB System/6
  assert_vld/1 -> MATLAB System/3
  deassert_lim/1 -> MATLAB System/4
  assert_lim/1 -> MATLAB System/2
  Rate Transition1/1 -> MATLAB System/1
  input/1 -> Rate Transition1/1
  Data Type Conversion/1 -> tfv_status/1
